simulink model "shift"  (R2018a)
settings: Solver=VariableStepAuto  StartTime=0.0  StopTime=10.0  RelTol=1e-3
settings Model: Creator=Edoardo Debenedetti  LastModifiedBy=Edoardo Debenedetti

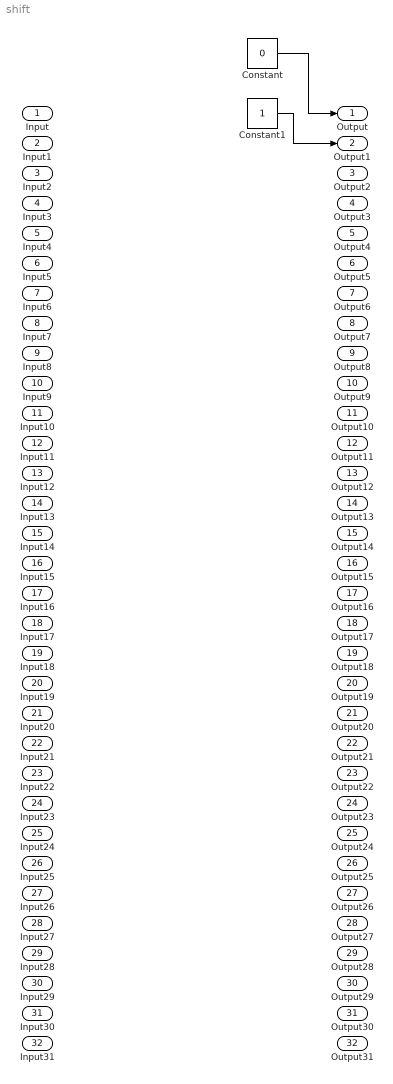
== system shift ==
  Input : Inport
  Input1 : Inport  Port=2
  Input2 : Inport  Port=3
  Input3 : Inport  Port=4
  Input4 : Inport  Port=5
  Input5 : Inport  Port=6
  Input6 : Inport  Port=7
  Input7 : Inport  Port=8
  Input8 : Inport  Port=9
  Input9 : Inport  Port=10
  Input10 : Inport  Port=11
  Input11 : Inport  Port=12
  Input12 : Inport  Port=13
  Input13 : Inport  Port=14
  Input14 : Inport  Port=15
  Input15 : Inport  Port=16
  Input16 : Inport  Port=17
  Input17 : Inport  Port=18
  Input18 : Inport  Port=19
  Input19 : Inport  Port=20
  Input20 : Inport  Port=21
  Input21 : Inport  Port=22
  Input22 : Inport  Port=23
  Input23 : Inport  Port=24
  Input24 : Inport  Port=25
  Input25 : Inport  Port=26
  Input26 : Inport  Port=27
  Input27 : Inport  Port=28
  Input28 : Inport  Port=29
  Input29 : Inport  Port=30
  Input30 : Inport  Port=31
  Input31 : Inport  Port=32
  Constant : Constant  Value=0
  Constant1 : Constant
  Output : Outport
  Output1 : Outport  Port=2
  Output2 : Outport  Port=3
  Output3 : Outport  Port=4
  Output4 : Outport  Port=5
  Output5 : Outport  Port=6
  Output6 : Outport  Port=7
  Output7 : Outport  Port=8
  Output8 : Outport  Port=9
  Output9 : Outport  Port=10
  Output10 : Outport  Port=11
  Output11 : Outport  Port=12
  Output12 : Outport  Port=13
  Output13 : Outport  Port=14
  Output14 : Outport  Port=15
  Output15 : Outport  Port=16
  Output16 : Outport  Port=17
  Output17 : Outport  Port=18
  Output18 : Outport  Port=19
  Output19 : Outport  Port=20
  Output20 : Outport  Port=21
  Output21 : Outport  Port=22
  Output22 : Outport  Port=23
  Output23 : Outport  Port=24
  Output24 : Outport  Port=25
  Output25 : Outport  Port=26
  Output26 : Outport  Port=27
  Output27 : Outport  Port=28
  Output28 : Outport  Port=29
  Output29 : Outport  Port=30
  Output30 : Outport  Port=31
  Output31 : Outport  Port=32
  wires:
  Constant/1 -> Output/1
  Constant1/1 -> Output1/1
